simulink model "ep_discrete"  (R2024b)
settings: Solver=VariableStepAuto  StartTime=0.0  StopTime=100  RelTol=1e-3
settings Model: Creator=merlin  LastModifiedBy=merlin

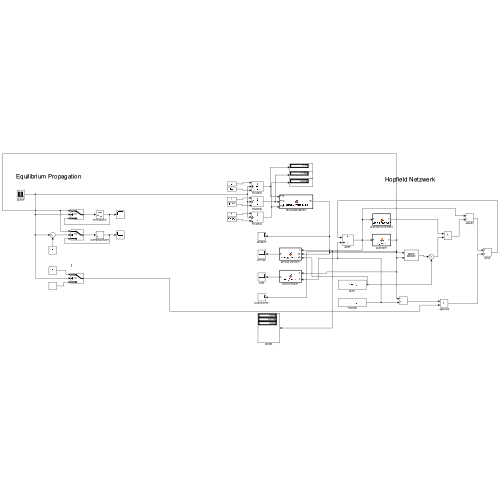
[thumbnail: Simulink's stored preview of the top-level diagram]
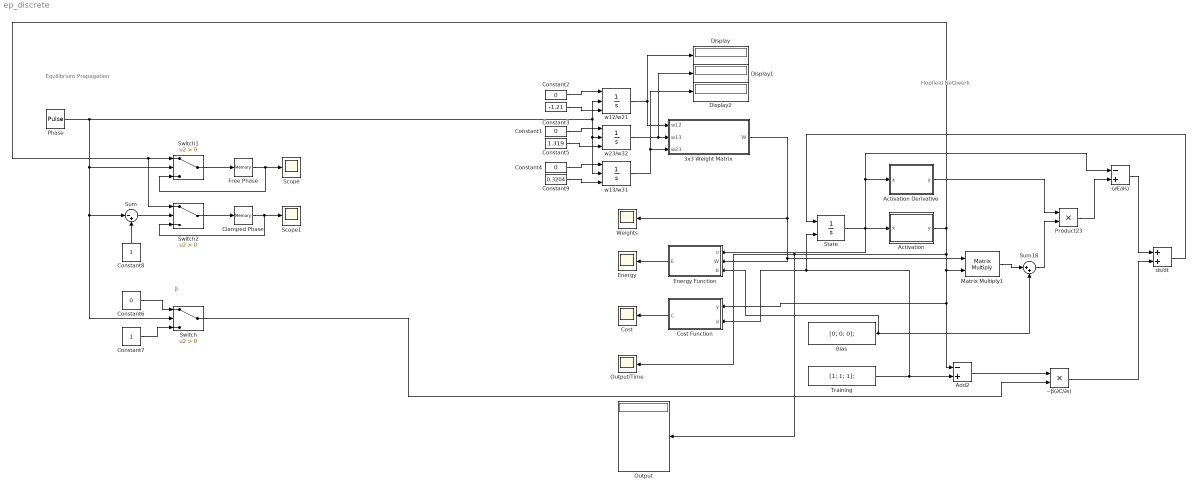
== system ep_discrete ==
  note: β
  note: Equilibrium Propagation
  note: Hopfield Netzwerk
  -(∂E/∂s) : Sum  Inputs=-+
  3x3 Weight Matrix : MATLAB Function  TreatAsAtomicUnit=on
  Activation : MATLAB Function  TreatAsAtomicUnit=on
  Activation Derivative : MATLAB Function  TreatAsAtomicUnit=on
  Add2 : Sum  Inputs=-+
  Bias : Constant  Value=[0; 0; 0];  VectorParams1D=off
  Clamped Phase : Memory
  Constant{1..2,4,6} (4 alike) : Constant  Value=0
  Constant3 : Constant  Value=-1.21
  Constant5 : Constant  Value=1.319
  Constant7 : Constant
  Constant8 : Constant
  Constant9 : Constant  Value=0.3204
  Cost : Scope
  Cost Function : MATLAB Function  TreatAsAtomicUnit=on
  Display : Display
  Display1 : Display
  Display2 : Display
  Energy : Scope
  Energy Function : MATLAB Function  TreatAsAtomicUnit=on
  Free Phase : Memory
  Matrix Multiply1 : Product  Multiplication=Matrix(*)
  Output : Display
  Output/Time : Scope
  Phase : DiscretePulseGenerator  PulseType=Time based  Period=20  PulseWidth=50
  Product23 : Product
  Scope : Scope
  Scope1 : Scope
  State : Integrator  InitialConditionSource=external
  Sum : Sum  Inputs=|-+
  Sum18 : Sum  Inputs=|++
  Switch : Switch  Criteria=u2 > Threshold  SaturateOnIntegerOverflow=off  InputSameDT=off
  Switch1 : Switch  Criteria=u2 > Threshold  SaturateOnIntegerOverflow=off  InputSameDT=off
  Switch2 : Switch  Criteria=u2 > Threshold  SaturateOnIntegerOverflow=off  InputSameDT=off
  Training : Constant  Value=[1; 1; 1];  VectorParams1D=off
  Weights : Scope
  ds/dt : Sum
  w12/w21 : Integrator  ExternalReset=either  InitialConditionSource=external
  w13/w31 : Integrator  ExternalReset=either  InitialConditionSource=external
  w23/w32 : Integrator  ExternalReset=either  InitialConditionSource=external
  −β(∂C/∂s) : Product
  wires:
  Constant6/1 -> Switch/1
  Constant7/1 -> Switch/3
  Phase/1 -> Switch1/2, Sum/1, Switch/2, w23/w32/2, w13/w31/2, w12/w21/2
  Constant8/1 -> Sum/2
  Sum/1 -> Switch2/2
  Switch1/1 -> Free Phase/1
  Switch2/1 -> Clamped Phase/1
  Free Phase/1 -> Switch1/3, Scope/1
  Clamped Phase/1 -> Switch2/3, Scope1/1
  Product23/1 -> -(∂E/∂s)/2
  Constant1/1 -> w23/w32/1
  Energy Function/1(E) -> Energy/1
  −β(∂C/∂s)/1 -> ds/dt/2
  Constant3/1 -> w12/w21/3
  Cost Function/1(C) -> Cost/1
  3x3 Weight Matrix/1(W) -> Weights/1, Energy Function/2(W), Matrix Multiply1/1
  w13/w31/1 -> Display2/1, 3x3 Weight Matrix/3(w23)
  Bias/1 -> Sum18/2, Energy Function/3(b)
  w12/w21/1 -> 3x3 Weight Matrix/1(w12), Display/1
  ds/dt/1 -> State/1
  Activation/1(y) -> Add2/1, Cost Function/1(y), Matrix Multiply1/2, Output/Time/1, Output/1, Switch2/1, Switch1/1
  Training/1 -> Cost Function/2(d), State/2, Add2/2
  Constant4/1 -> w13/w31/1
  -(∂E/∂s)/1 -> ds/dt/1
  State/1 -> Activation/1(x), Energy Function/1(u), Activation Derivative/1(x), -(∂E/∂s)/1
  w23/w32/1 -> Display1/1, 3x3 Weight Matrix/2(w13)
  Add2/1 -> −β(∂C/∂s)/1
  Constant9/1 -> w13/w31/3
  Sum18/1 -> Product23/2
  Constant5/1 -> w23/w32/3
  Matrix Multiply1/1 -> Sum18/1
  Constant2/1 -> w12/w21/1
  Activation Derivative/1(y) -> Product23/1
  Switch/1 -> −β(∂C/∂s)/2

== matlab function ep_discrete/3x3 Weight Matrix ==
  data: w12 input; W output; w13 input; w23 input
function W = create3x3WeightMatrix(w12, w13, w23)
    W = [0,    w12,  w13;
         w12,  0,    w23;
         w13,  w23,  0];
end

== matlab function ep_discrete/Energy Function ==
  data: u input; E output; W input; b input
function E = energy_function(u, W, b)
    rho = @(x) 1 ./ (1 + exp(-x));

    E = (1/2) * sum(u.^2) ...
        - (1/2) * sum(sum(W .* (rho(u) * rho(u)')))
        - sum(b .* rho(u));
end

== matlab function ep_discrete/Activation Derivative ==
  data: x input; y output
function y = sigmoid_derivative(x)
sigmoid = 1 ./ (1 + exp(-x));
y = sigmoid .* (1 - sigmoid);
end

== matlab function ep_discrete/Activation ==
  data: x input; y output
function y = sigmoid(x)
y = 1 ./ (1 + exp(-x));
end

== matlab function ep_discrete/Cost Function ==
  data: y input; C output; d input
function C = cost_function(y, d)
    C = 0.5 * sum((y - d).^2);
end
